simulink subsystem "CAN"  (R2022b)
settings: Solver=VariableStepAuto  StartTime=0.0  StopTime=10.0  RelTol=1e-3
libraries: Raptor_lib x4
settings Model: Creator=serga  LastModifiedBy=serga

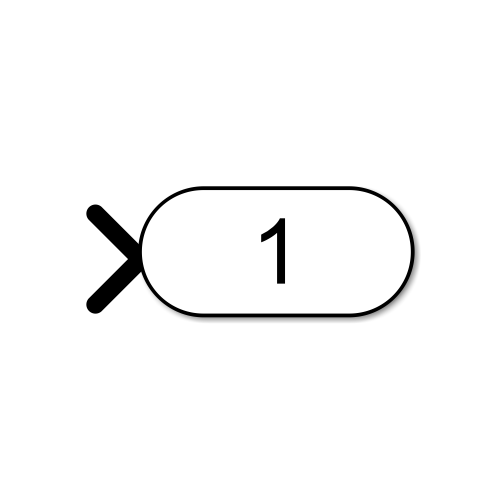
[thumbnail: Simulink's stored preview of the top-level diagram]
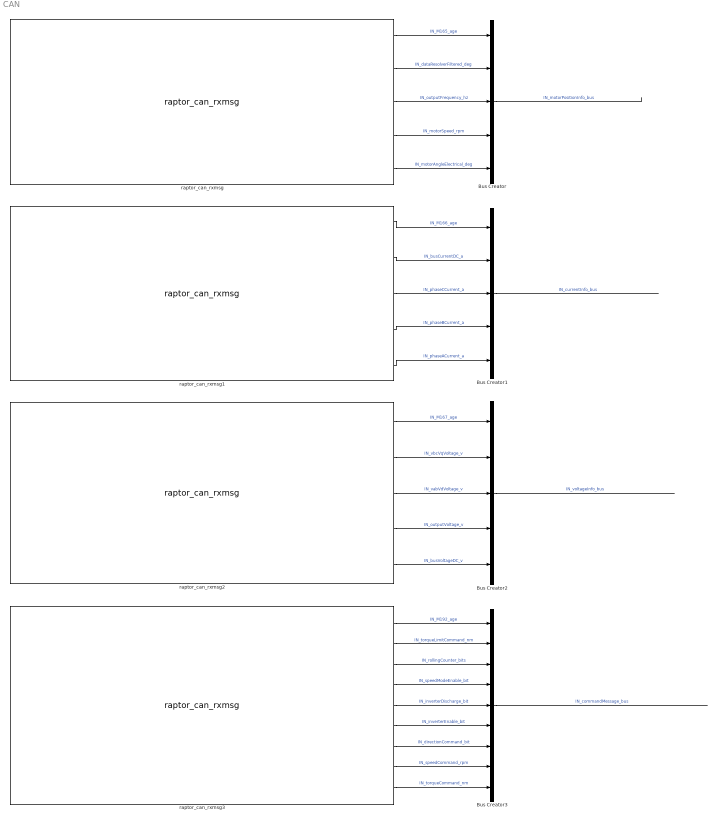
== system CAN ==
  Bus Creator : BusCreator  Inputs=5
  Bus Creator1 : BusCreator  Inputs=5
  Bus Creator2 : BusCreator  Inputs=5
  Bus Creator3 : BusCreator  Inputs=9
  raptor_can_rxmsg : Raptor_lib/CAN/raptor_can_rxmsg  canDefinition=struct('dbcFile', 'inverterCAN.dbc','message', 'M165_Motor_Position_Info','comment', '','signals', {{'D4_Delta_Resolver_Filtered','D3_Electrical_Output_Frequency','D2_Motor_Speed','D1_Motor_Angle_Electrical'}},'enabled', [ 1 1 1 1;],'scaled', [ 1 1 1 1;],'canBus', '''CAN1''','messageID', [ 165;],'idMask', [ 536870911;],'payloadMask', [],'payloadValue', [],'period', [ 0;],'mailbox', '''''','queueSize', [ 1;],'label', [ 0;],'ver', [ 2;],'showID', [ 0;],'showRaw', [ 0;],'showRawMsg', [ 0;],'useStartVals', [ 0;],'showAge', [ 1;],'useSimFunc', [ 0;],'sim_func_name', '''''','fill', [ 0;],'editID', [ 0;],'signalOrder', [ 2;],'signalAscDes', [ 1;],'msgLength', [ 8;])  canBus='CAN1'  mailbox=''  payloadMask=[]  payloadValue=[]  idMask=hex2dec('1FFFFFFF')  queueSize=1  showID=0  label=0  fill=0  id=165  showRaw=0  showAge=1  signalOrder=2  signalInfo={{struct('Name', 'D4_Delta_Resolver_Filtered','StartBit', [ 48;],'SignalSize', [ 16;],'ByteOrder', 'LittleEndian','ValueType', 'SIGNED','Class', 'int16','Signed', [ 1;],'Factor', [ 0.1;],'Offset', [ 0;],'Min', [ -3276.8;],'Max', [ 3276.7;],'Units', 'deg','StartVal', [ 0;],'Comment', 'Used in calibration of resolver angle adjustment.','Multiplexed', [ 0;],'Multiplexor', [ 0;],'MultiplexMode_Min', [ 0;],'MultiplexMode_Max', [ 0;]),struct('Name', 'D3_Electrical_Output_Frequency','StartBit', [ 32;],'SignalSize', [ 16;],'ByteOrder', 'LittleEndian','ValueType', 'SIGNED','Class', 'int16','Signed', [ 1;],'Factor', [ 0.1;],'Offset', [ 0;],'Min', [ -3276.8;],'Max', [ 3276.7;],'Units', 'hz','StartVal', [ 0;],'Comment', 'The actual electrical frequency of the inverter','Multiplexed', [ 0;],'Multiplexor', [ 0;],'MultiplexMode_Min', [ 0;],'MultiplexMode_Max', [ 0;]),struct('Name', 'D2_Motor_Speed','StartBit', [ 16;],'SignalSize', [ 16;],'ByteOrder', 'LittleEndian','ValueType', 'SIGNED','Class', 'int16','Signed', [ 1;],'Factor', [ 1;],'Offset', [ 0;],'Min', [ -32768;],'Max', [ 32767;],'Units', 'rpm','StartVal', [ 0;],'Comment', 'The measured speed of the motor','Multiplexed', [ 0;],'Multiplexor', [ 0;],'MultiplexMode_Min', [ 0;],'MultiplexMode_Max', [ 0;]),struct('Name', 'D1_Motor_Angle_Electrical','StartBit', [ 0;],'SignalSize', [ 16;],'ByteOrder', 'LittleEndian','ValueType', 'UNSIGNED','Class', 'uint16','Signed', [ 0;],'Factor', [ 0.1;],'Offset', [ 0;],'Min', [ 0;],'Max', [ 6553.5;],'Units', 'deg','StartVal', [ 0;],'Comment', 'The Electrical Angle of the motor as read by the encoder or resolver','Multiplexed', [ 0;],'Multiplexor', [ 0;],'MultiplexMode_Min', [ 0;],'MultiplexMode_Max', [ 0;])}}  showRawMsg=0  useSimFunc=0  sim_func_name=''  useStartVals=0
      settings: SourceProductName=Raptor
  raptor_can_rxmsg1 : Raptor_lib/CAN/raptor_can_rxmsg  canDefinition=struct('dbcFile', 'inverterCAN.dbc','message', 'M166_Current_Info','comment', '','signals', {{'D4_DC_Bus_Current','D3_Phase_C_Current','D2_Phase_B_Current','D1_Phase_A_Current'}},'enabled', [ 1 1 1 1;],'scaled', [ 1 1 1 1;],'canBus', '''CAN1''','messageID', [ 166;],'idMask', [ 536870911;],'payloadMask', [],'payloadValue', [],'period', [ 0;],'mailbox', '''''','queueSize', [ 1;],'label', [ 0;],'ver', [ 2;],'showID', [ 0;],'showRaw', [ 0;],'showRawMsg', [ 0;],'useStartVals', [ 0;],'showAge', [ 1;],'useSimFunc', [ 0;],'sim_func_name', '''''','fill', [ 0;],'editID', [ 0;],'signalOrder', [ 2;],'signalAscDes', [ 1;],'msgLength', [ 8;])  canBus='CAN1'  mailbox=''  payloadMask=[]  payloadValue=[]  idMask=hex2dec('1FFFFFFF')  queueSize=1  showID=0  label=0  fill=0  id=166  showRaw=0  showAge=1  signalOrder=2  signalInfo={{struct('Name', 'D4_DC_Bus_Current','StartBit', [ 48;],'SignalSize', [ 16;],'ByteOrder', 'LittleEndian','ValueType', 'SIGNED','Class', 'int16','Signed', [ 1;],'Factor', [ 0.1;],'Offset', [ 0;],'Min', [ -3276.8;],'Max', [ 3276.7;],'Units', 'A','StartVal', [ 0;],'Comment', 'The Calculated DC Bus Current','Multiplexed', [ 0;],'Multiplexor', [ 0;],'MultiplexMode_Min', [ 0;],'MultiplexMode_Max', [ 0;]),struct('Name', 'D3_Phase_C_Current','StartBit', [ 32;],'SignalSize', [ 16;],'ByteOrder', 'LittleEndian','ValueType', 'SIGNED','Class', 'int16','Signed', [ 1;],'Factor', [ 0.1;],'Offset', [ 0;],'Min', [ -3276.8;],'Max', [ 3276.7;],'Units', 'A','StartVal', [ 0;],'Comment', 'The measured value of Phase C current','Multiplexed', [ 0;],'Multiplexor', [ 0;],'MultiplexMode_Min', [ 0;],'MultiplexMode_Max', [ 0;]),struct('Name', 'D2_Phase_B_Current','StartBit', [ 16;],'SignalSize', [ 16;],'ByteOrder', 'LittleEndian','ValueType', 'SIGNED','Class', 'int16','Signed', [ 1;],'Factor', [ 0.1;],'Offset', [ 0;],'Min', [ -3276.8;],'Max', [ 3276.7;],'Units', 'A','StartVal', [ 0;],'Comment', 'The measured value of Phase B current','Multiplexed', [ 0;],'Multiplexor', [ 0;],'MultiplexMode_Min', [ 0;],'MultiplexMode_Max', [ 0;]),struct('Name', 'D1_Phase_A_Current','StartBit', [ 0;],'SignalSize', [ 16;],'ByteOrder', 'LittleEndian','ValueType', 'SIGNED','Class', 'int16','Signed', [ 1;],'Factor', [ 0.1;],'Offset', [ 0;],'Min', [ -3276.8;],'Max', [ 3276.7;],'Units', 'A','StartVal', [ 0;],'Comment', 'The measured value of Phase A current','Multiplexed', [ 0;],'Multiplexor', [ 0;],'MultiplexMode_Min', [ 0;],'MultiplexMode_Max', [ 0;])}}  showRawMsg=0  useSimFunc=0  sim_func_name=''  useStartVals=0
      settings: SourceProductName=Raptor
  raptor_can_rxmsg2 : Raptor_lib/CAN/raptor_can_rxmsg  canDefinition=struct('dbcFile', 'inverterCAN.dbc','message', 'M167_Voltage_Info','comment', '','signals', {{'D4_VBC_Vq_Voltage','D3_VAB_Vd_Voltage','D2_Output_Voltage','D1_DC_Bus_Voltage'}},'enabled', [ 1 1 1 1;],'scaled', [ 1 1 1 1;],'canBus', '''CAN1''','messageID', [ 167;],'idMask', [ 536870911;],'payloadMask', [],'payloadValue', [],'period', [ 0;],'mailbox', '''''','queueSize', [ 1;],'label', [ 0;],'ver', [ 2;],'showID', [ 0;],'showRaw', [ 0;],'showRawMsg', [ 0;],'useStartVals', [ 0;],'showAge', [ 1;],'useSimFunc', [ 0;],'sim_func_name', '''''','fill', [ 0;],'editID', [ 0;],'signalOrder', [ 2;],'signalAscDes', [ 1;],'msgLength', [ 8;])  canBus='CAN1'  mailbox=''  payloadMask=[]  payloadValue=[]  idMask=hex2dec('1FFFFFFF')  queueSize=1  showID=0  label=0  fill=0  id=167  showRaw=0  showAge=1  signalOrder=2  signalInfo={{struct('Name', 'D4_VBC_Vq_Voltage','StartBit', [ 48;],'SignalSize', [ 16;],'ByteOrder', 'LittleEndian','ValueType', 'SIGNED','Class', 'int16','Signed', [ 1;],'Factor', [ 0.1;],'Offset', [ 0;],'Min', [ -3276.8;],'Max', [ 3276.7;],'Units', 'V','StartVal', [ 0;],'Comment', 'Measured value of the voltage between Phase B and Phase C','Multiplexed', [ 0;],'Multiplexor', [ 0;],'MultiplexMode_Min', [ 0;],'MultiplexMode_Max', [ 0;]),struct('Name', 'D3_VAB_Vd_Voltage','StartBit', [ 32;],'SignalSize', [ 16;],'ByteOrder', 'LittleEndian','ValueType', 'SIGNED','Class', 'int16','Signed', [ 1;],'Factor', [ 0.1;],'Offset', [ 0;],'Min', [ -3276.8;],'Max', [ 3276.7;],'Units', 'V','StartVal', [ 0;],'Comment', 'Measured value of the voltage betwen phase A and Phase B','Multiplexed', [ 0;],'Multiplexor', [ 0;],'MultiplexMode_Min', [ 0;],'MultiplexMode_Max', [ 0;]),struct('Name', 'D2_Output_Voltage','StartBit', [ 16;],'SignalSize', [ 16;],'ByteOrder', 'LittleEndian','ValueType', 'SIGNED','Class', 'int16','Signed', [ 1;],'Factor', [ 0.1;],'Offset', [ 0;],'Min', [ -3276.8;],'Max', [ 3276.7;],'Units', 'V','StartVal', [ 0;],'Comment', 'The calculated value of the output voltage, in peak line-neutral volts','Multiplexed', [ 0;],'Multiplexor', [ 0;],'MultiplexMode_Min', [ 0;],'MultiplexMode_Max', [ 0;]),struct('Name', 'D1_DC_Bus_Voltage','StartBit', [ 0;],'SignalSize', [ 16;],'ByteOrder', 'LittleEndian','ValueType', 'SIGNED','Class', 'int16','Signed', [ 1;],'Factor', [ 0.1;],'Offset', [ 0;],'Min', [ -3276.8;],'Max', [ 3276.7;],'Units', 'V','StartVal', [ 0;],'Comment', 'The actual measured value of the DC bus voltage','Multiplexed', [ 0;],'Multiplexor', [ 0;],'MultiplexMode_Min', [ 0;],'MultiplexMode_Max', [ 0;])}}  showRawMsg=0  useSimFunc=0  sim_func_name=''  useStartVals=0
      settings: SourceProductName=Raptor
  raptor_can_rxmsg3 : Raptor_lib/CAN/raptor_can_rxmsg  canDefinition=struct('dbcFile', 'inverterCAN.dbc','message', 'M192_Command_Message','comment', 'The command message is used to transmit data to the controller. This message is sent from a user supplied external controller to the PMxxx controller.','signals', {{'Torque_Limit_Command','RollingCounter','Speed_Mode_Enable','Inverter_Discharge','Inverter_Enable','Direction_Command','Speed_Command','Torque_Command'}},'enabled', [ 1 1 1 1 1 1 1 1;],'scaled', [ 1 1 1 1 1 1 1 1;],'canBus', '''CAN1''','messageID', [ 192;],'idMask', [ 536870911;],'payloadMask', [],'payloadValue', [],'period', [ 0;],'mailbox', '''''','queueSize', [ 1;],'label', [ 0;],'ver', [ 2;],'showID', [ 0;],'showRaw', [ 0;],'showRawMsg', [ 0;],'useStartVals', [ 0;],'showAge', [ 1;],'useSimFunc', [ 0;],'sim_func_name', '''''','fill', [ 0;],'editID', [ 0;],'signalOrder', [ 2;],'signalAscDes', [ 1;],'msgLength', [ 8;])  canBus='CAN1'  mailbox=''  payloadMask=[]  payloadValue=[]  idMask=hex2dec('1FFFFFFF')  queueSize=1  showID=0  label=0  fill=0  id=192  showRaw=0  showAge=1  signalOrder=2  signalInfo={{struct('Name', 'Inverter_Enable','StartBit', [ 40;],'SignalSize', [ 1;],'ByteOrder', 'LittleEndian','ValueType', 'UNSIGNED','Class', 'uint8','Signed', [ 0;],'Factor', [ 1;],'Offset', [ 0;],'Min', [ 0;],'Max', [ 1;],'Units', 'Bit','StartVal', [ 0;],'Comment', '0=Inverter OFF, 1 = Inverter ON','Multiplexed', [ 0;],'Multiplexor', [ 0;],'MultiplexMode_Min', [ 0;],'MultiplexMode_Max', [ 0;]),struct('Name', 'Direction_Command','StartBit', [ 32;],'SignalSize', [ 1;],'ByteOrder', 'LittleEndian','ValueType', 'UNSIGNED','Class', 'uint8','Signed', [ 0;],'Factor', [ 1;],'Offset', [ 0;],'Min', [ 0;],'Max', [ 1;],'Units', 'Bit','StartVal', [ 0;],'Comment', '0=CW, 1=CCW as veiwed from the shaft end of the motor','Multiplexed', [ 0;],'Multiplexor', [ 0;],'MultiplexMode_Min', [ 0;],'MultiplexMode_Max', [ 0;]),struct('Name', 'Speed_Command','StartBit', [ 16;],'SignalSize', [ 16;],'ByteOrder', 'LittleEndian','ValueType', 'SIGNED','Class', 'int16','Signed', [ 1;],'Factor', [ 1;],'Offset', [ 0;],'Min', [ -32768;],'Max', [ 32767;],'Units', 'rpm','StartVal', [ 0;],'Comment', 'Speed commandused when in speed mode','Multiplexed', [ 0;],'Multiplexor', [ 0;],'MultiplexMode_Min', [ 0;],'MultiplexMode_Max', [ 0;]),struct('Name', 'Torque_Command','StartBit', [ 0;],'SignalSize', [ 16;],'ByteOrder', 'LittleEndian','ValueType', 'SIGNED','Class', 'int16','Signed', [ 1;],'Factor', [ 0.1;],'Offset', [ 0;],'Min', [ -3276.8;],'Max', [ 3276.7;],'Units', 'Nm','StartVal', [ 0;],'Comment', 'Torque command when in torque mode','Multiplexed', [ 0;],'Multiplexor', [ 0;],'MultiplexMode_Min', [ 0;],'MultiplexMode_Max', [ 0;]),struct('Name', 'Inverter_Discharge','StartBit', [ 41;],'SignalSize', [ 1;],'ByteOrder', 'LittleEndian','ValueType', 'UNSIGNED','Class', 'uint8','Signed', [ 0;],'Factor', [ 1;],'Offset', [ 0;],'Min', [ 0;],'Max', [ 1;],'Units', 'Bit','StartVal', [ 0;],'Comment', '0=Discharge Disable,','Multiplexed', [ 0;],'Multiplexor', [ 0;],'MultiplexMode_Min', [ 0;],'MultiplexMode_Max', [ 0;]),struct('Name', 'Torque_Limit_Command','StartBit', [ 48;],'SignalSize', [ 16;],'ByteOrder', 'LittleEndian','ValueType', 'SIGNED','Class', 'int16','Signed', [ 1;],'Factor', [ 0.1;],'Offset', [ 0;],'Min', [ -3276.8;],'Max', [ 3276.7;],'Units', 'Nm','StartVal', [ 0;],'Comment', 'Torque Limit, set to 0 to keep default','Multiplexed', [ 0;],'Multiplexor', [ 0;],'MultiplexMode_Min', [ 0;],'MultiplexMode_Max', [ 0;]),struct('Name', 'Speed_Mode_Enable','StartBit', [ 42;],'SignalSize', [ 1;],'ByteOrder', 'LittleEndian','ValueType', 'UNSIGNED','Class', 'uint8','Signed', [ 0;],'Factor', [ 1;],'Offset', [ 0;],'Min', [ 0;],'Max', [ 1;],'Units', 'Bit','StartVal', [ 0;],'Comment', '0 = No change to mode, 1 = change to speed mode from torque mode','Multiplexed', [ 0;],'Multiplexor', [ 0;],'MultiplexMode_Min', [ 0;],'MultiplexMode_Max', [ 0;]),struct('Name', 'RollingCounter','StartBit', [ 44;],'SignalSize', [ 4;],'ByteOrder', 'LittleEndian','ValueType', 'UNSIGNED','Class', 'uint8','Signed', [ 0;],'Factor', [ 1;],'Offset', [ 0;],'Min', [ 0;],'Max', [ 15;],'Units', 'Bits','StartVal', [ 0;],'Comment', 'Rolling Counter command','Multiplexed', [ 0;],'Multiplexor', [ 0;],'MultiplexMode_Min', [ 0;],'MultiplexMode_Max', [ 0;])}}  showRawMsg=0  useSimFunc=0  sim_func_name=''  useStartVals=0
      settings: SourceProductName=Raptor
  wires:
  raptor_can_rxmsg/1 -> Bus Creator/1  "IN_M165_age"
  raptor_can_rxmsg/2 -> Bus Creator/2  "IN_dataResolverFiltered_deg"
  raptor_can_rxmsg/3 -> Bus Creator/3  "IN_outputFrequency_hz"
  raptor_can_rxmsg/5 -> Bus Creator/5  "IN_motorAngleElectrical_deg"
  raptor_can_rxmsg/4 -> Bus Creator/4  "IN_motorSpeed_rpm"
  raptor_can_rxmsg1/2 -> Bus Creator1/2  "IN_busCurrentDC_a"
  raptor_can_rxmsg1/1 -> Bus Creator1/1  "IN_M166_age"
  raptor_can_rxmsg1/3 -> Bus Creator1/3  "IN_phaseCCurrent_a"
  raptor_can_rxmsg1/4 -> Bus Creator1/4  "IN_phaseBCurrent_a"
  raptor_can_rxmsg1/5 -> Bus Creator1/5  "IN_phaseACurrent_a"
  Bus Creator/1 -> ?  "IN_motorPositionInfo_bus"
  Bus Creator1/1 -> ?  "IN_currentInfo_bus"
  raptor_can_rxmsg2/3 -> Bus Creator2/3  "IN_vabVdVoltage_v"
  raptor_can_rxmsg2/2 -> Bus Creator2/2  "IN_vbcVqVoltage_v"
  raptor_can_rxmsg2/1 -> Bus Creator2/1  "IN_M167_age"
  raptor_can_rxmsg2/4 -> Bus Creator2/4  "IN_outputVoltage_v"
  raptor_can_rxmsg2/5 -> Bus Creator2/5  "IN_busVoltageDC_v"
  Bus Creator2/1 -> ?  "IN_voltageInfo_bus"
  raptor_can_rxmsg3/1 -> Bus Creator3/1  "IN_M192_age"
  raptor_can_rxmsg3/2 -> Bus Creator3/2  "IN_torqueLimitCommand_nm"
  raptor_can_rxmsg3/3 -> Bus Creator3/3  "IN_rollingCounter_bits"
  raptor_can_rxmsg3/4 -> Bus Creator3/4  "IN_speedModeEnable_bit"
  raptor_can_rxmsg3/5 -> Bus Creator3/5  "IN_inverterDischarge_bit"
  raptor_can_rxmsg3/6 -> Bus Creator3/6  "IN_inverterEnable_bit"
  raptor_can_rxmsg3/7 -> Bus Creator3/7  "IN_directionCommand_bit"
  raptor_can_rxmsg3/8 -> Bus Creator3/8  "IN_speedCommand_rpm"
  raptor_can_rxmsg3/9 -> Bus Creator3/9  "IN_torqueCommand_nm"
  Bus Creator3/1 -> ?  "IN_commandMessage_bus"
